simulink model "conlac1"  (Simulink 7.4)
settings: Solver=ode45  StartTime=0.0  StopTime=10.0  RelTol=1e-3
settings Model: Creator=phuck  LastModifiedBy=phuck

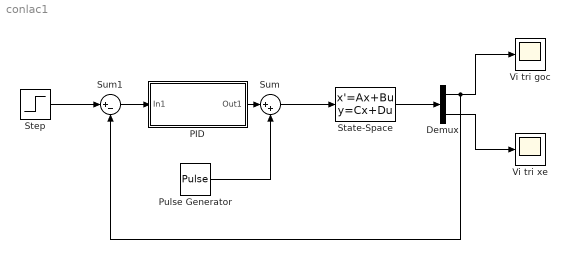
== system conlac1 ==
  Demux : Demux  Outputs=2
  PID : Subsystem
  Pulse Generator : DiscretePulseGenerator  PulseType=Time based  Amplitude=1  Period=10  PulseWidth=5  PhaseDelay=0  SampleTime=1
  State-Space : StateSpace  A=[0 1.0000 0 0;15.7756 0 0 0;0 0 0 1.0000;-0.7171 0 0 0]  B=[0;-1.4634;0;0.9756]  C=[1 0 0 0;0 0 1 0]  D=[0;0]
  Step : Step  Time=0  SampleTime=0
  Sum : Sum  Inputs=|++  OutDataType=fixdt(1, 16)  OutScaling=2^0
  Sum1 : Sum  Inputs=|+-  OutDataType=fixdt(1, 16)  OutScaling=2^0
  Vi tri goc : Scope
  Vi tri xe : Scope
  wires:
  Demux/1 -> Vi tri goc/1, Sum1/2
  Demux/2 -> Vi tri xe/1
  State-Space/1 -> Demux/1
  Pulse Generator/1 -> Sum/2
  Sum/1 -> State-Space/1
  Step/1 -> Sum1/1
  Sum1/1 -> PID/1(In1)
  PID/1(Out1) -> Sum/1

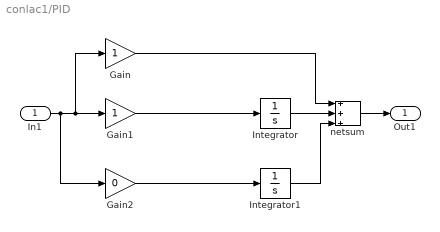
== system conlac1/PID ==
  In1 : Inport  OutDataType=fixdt(1, 16)  OutScaling=2^0
  Gain : Gain  ParameterDataType=fixdt(1, 16)  ParameterScaling=2^0  OutDataType=fixdt(1, 16)  OutScaling=2^0
  Gain1 : Gain  ParameterDataType=fixdt(1, 16)  ParameterScaling=2^0  OutDataType=fixdt(1, 16)  OutScaling=2^0
  Gain2 : Gain  Gain=0  ParameterDataType=fixdt(1, 16)  ParameterScaling=2^0  OutDataType=fixdt(1, 16)  OutScaling=2^0
  Integrator : Integrator
  Integrator1 : Integrator
  netsum : Sum  Inputs=3  OutDataType=sfix(16)  OutScaling=2^0  SaturateOnIntegerOverflow=on  InputSameDT=on  OutDataTypeStr=Inherit: Same as first input
  Out1 : Outport  OutDataType=fixdt(1, 16)  OutScaling=2^0
  wires:
  In1/1 -> Gain1/1, Gain/1, Gain2/1
  Gain/1 -> netsum/1
  Gain1/1 -> Integrator/1
  Integrator/1 -> netsum/2
  netsum/1 -> Out1/1
  Integrator1/1 -> netsum/3
  Gain2/1 -> Integrator1/1
